simulink model "EnvironmentalControlSystem"  (R2018b)
settings: Solver=FixedStepAuto  StartTime=0.0  StopTime=500  FixedStep=0.01  RelTol=1e-3
values from neighbouring files (symbols this model uses):
  dt = 0.01    [run_sim.m]    (also in sys_id_pipeline.m = mean(diff(Time_vec_full)))
  K31 = Result31.K_slope    [sys_id_pipeline.m]
  K32 = Result32.K_slope    [sys_id_pipeline.m]
  P_ref = GlobalParams.P_ref    [sys_id_pipeline.m]
  Patm = GlobalParams.Patm    [sys_id_pipeline.m]
  R_gas = GlobalParams.R    [sys_id_pipeline.m]
  T_ref = GlobalParams.T_ref    [sys_id_pipeline.m]
  Tau31 = 5    [sys_id_pipeline.m]
  Tau32 = 5    [sys_id_pipeline.m]
  Tp31 = Result31.Tp    [sys_id_pipeline.m]
  Tp32 = Result32.Tp    [sys_id_pipeline.m]
  V_vol = pi * (0.05)^2 * 5    (= 0.0392699081699)    [run_sim.m]
  X31_den = sys_X31.Denominator    [sys_id_value.m]
  X31_num = sys_X31.Numerator    [sys_id_value.m]
  X32_den = sys_X32.Denominator    [sys_id_value.m]
  X32_num = sys_X32.Numerator    [sys_id_value.m]
libraries: simulink x14
(part 3 of 3)

== matlab function EnvironmentalControlSystem/ECS Controller/Smith_PI_Controller/Smith_PI_Controller ==
  settings: updateMethod=DISCRETE
  data: Q31Ref input; V31 output; Q31Real input; Q32Ref input; Q32Real input; P30 input; T30 input; V32 output; K31 parameter; Tau31 parameter; K32 parameter; Tau32 parameter; P_ref parameter; T_ref parameter; R_gas parameter; Patm parameter; X31_num parameter; X31_den parameter; X32_num parameter; Tp31 parameter; X32_den parameter; Tp32 parameter
function [V31, V32] = Smith_PI_Controller(Q31Ref, Q31Real, Q32Ref, Q32Real, P30, T30, K31, Tau31, K32, Tau32, P_ref, T_ref, R_gas, Patm, X31_num, X31_den, X32_num, Tp31, X32_den, Tp32)
    % Smith_PI_Controller_Optimized
    %
    % 本函数实现了一种针对双通道非线性流量控制系统的优化 Smith 预估 PI 控制策略。
    % 针对两路子系统（Q31和Q32）显著不同的动态特性（过阻尼 vs 欠阻尼）以及共同存在的
    % 执行器死区（Actuator Deadzone）和纯滞后（Pure Time Delay）问题，
    % 采用了差异化的控制律设计。核心算法集成了基于内部模型的 Smith 预估器以补偿滞后，
    % 并引入了动态软死区补偿（Soft Deadzone Compensation）、抗积分饱和（Anti-windup）
    % 以及软件误差死区（Software Error Deadband）机制，以解决响应迟滞和极限环震荡（Limit Cycle Oscillation）问题。
    %
    % 系统特性描述 (System Characterization):
    % 1. 通道 Q31 (过阻尼 Over-damped):
    %    - 特性：大惯性，响应迟钝，存在显著静摩擦。
    %    - 问题：起步困难，稳态易受死区补偿过度影响产生等幅震荡。
    %    - 策略：采用高增益 Smith-PI 进行快速驱动，结合带锁存功能的软死区补偿，以及较宽的误差死区来抑制稳态打桩效应。
    %
    % 2. 通道 Q32 (欠阻尼 Under-damped):
    %    - 特性：响应灵敏，阻尼比小，易超调。
    %    - 问题：系统本身接近临界稳定，易诱发高频震荡和极限环。
    %    - 策略：采用低增益控制，配合强效的软件误差死区，在稳态时切断积分作用，消除震荡源。
    %
    % 输入变量定义 (Input Variables):
    %   Q31Ref, Q32Ref : 流量设定值 (Reference Setpoint) [kg/h]
    %   Q31Real, Q32Real: 流量过程变量 (Process Variable) [kg/h]
    %   P30            : 上游压力 (Upstream Pressure) [kPa]
    %   T30            : 上游温度 (Upstream Temperature) [degC]
    %   [模型参数]      : K(静态增益), Tau(纯滞后), X_num/den(阀门传递函数系数), Tp(时间常数)
    %
    % 输出变量定义 (Output Variables):
    %   V31, V32       : 阀门控制指令 (Control Variable) [0-100%]

    % === 1. 状态记忆区 (Persistent State Memory) ===
    % 用于离散时间控制系统的状态保持
    
    persistent integrator_31 integrator_32  % PI控制器积分项累加器
    persistent model_31 model_32            % 内部快速模型状态向量 [阀位 x1; 阀速 x2; 流量 x3]
    persistent delay_buffer_31 delay_buffer_32 % 环形缓冲区，用于模拟纯滞后 Tau
    persistent head_31 head_32              % 环形缓冲区写指针
    persistent u_prev_31 u_prev_32          % 上一控制周期的输出指令 (用于差分计算)
    persistent first_run                    % 初始化标志位
    
    MAX_BUF = 1000; % 缓冲区最大长度 (支持的最大滞后步数)

    % === 系统初始化 (System Initialization) ===
    if isempty(first_run)
        integrator_31 = 0; integrator_32 = 0;
        model_31 = [0;0;0]; model_32 = [0;0;0];
        delay_buffer_31 = zeros(MAX_BUF, 1);
        delay_buffer_32 = zeros(MAX_BUF, 1);
        head_31 = 1; head_32 = 1;
        u_prev_31 = 0; u_prev_32 = 0;
        first_run = 0;
    end

    % === 2. 全局参数设定 (Global Parameters) ===
    Ts = 0.01; % 采样周期 (Sample Time) [s]
    
    % 增益调度因子计算 (Gain Scheduling Factor)
    % 依据流体力学原理，流量与压差平方根成正比。通过 Ratio 归一化过程增益，
    % 使得控制器在不同工况下保持一致的环路增益。
    Ratio = CalculateFlowRatio(P30, T30, P_ref, T_ref, R_gas, Patm);

    % ==========================================================
    %       控制策略配置 (CONTROL STRATEGY CONFIGURATION)
    % ==========================================================

    % --- 通道 31 配置 (针对过阻尼系统) ---
    % 策略逻辑：
    % 1. Kp_31 (1.8): 设置较高比例增益。Smith 预估器消除了滞后导致的相位滞后，允许提高带宽以克服过阻尼系统的惯性。
    % 2. Ti_31 (2.5): 增大积分时间常数。减弱积分作用，防止积分器在死区边缘过度充能，导致系统在目标值附近反复超调。
    % 3. Gap_31 (1.4): 适中的死区补偿值。用于在指令变化时提供额外的“启动脉冲”，克服静摩擦力。
    % 4. Err_Band_31 (0.6): 较宽的误差死区。这是消除稳态等幅震荡（Limit Cycle）的关键。当误差进入此范围，控制器停止调节，避免微小扰动触发死区补偿。
    Kp_31 = 1.8;  
    Ti_31 = 25;  
    Gap_31 = 1.4; 
    Err_Band_31 = 0.6; 

    % --- 通道 32 配置 (针对欠阻尼系统) ---
    % 策略逻辑：
    % 1. Kp_32 (0.3): 设置较低比例增益。欠阻尼系统对激励敏感，高增益极易激发系统固有频率震荡。
    % 2. Ti_32 (5.0): 极大的积分时间常数。微弱的积分作用仅用于消除长期静差，防止诱发过冲。
    % 3. Gap_32 (0.6): 较小的死区补偿。欠阻尼系统惯性小，无需强力启动，过大补偿会导致响应过激。
    % 4. Err_Band_32 (0.8): 宽误差死区。欠阻尼系统难以精确稳定在零误差，宽死区相当于提供一个“稳定停泊区”，切断极限环。
    Kp_32 = 0.3;  
    Ti_32 = 8.0;  
    Gap_32 = 0.6; 
    Err_Band_32 = 0.1; 

    % ==========================================================

    % --- 自适应控制参数计算 (Adaptive Parameter Calculation) ---
    % 根据当前的物理工况 (Ratio) 实时调整 PI 参数
    Ki_31 = Kp_31 / Ti_31;
    Kp_31_adpt = Kp_31 / Ratio;
    Ki_31_adpt = Ki_31 / Ratio;
    
    Ki_32 = Kp_32 / Ti_32;
    Kp_32_adpt = Kp_32 / Ratio;
    Ki_32_adpt = Ki_32 / Ratio;

    % ==========================================================
    %       通道 31 控制回路执行 (Control Loop Execution - Ch31)
    % ==========================================================
    
    % 1. Smith 预估器模型更新
    % 这里的模型不包含纯滞后，用于预测当前的“虚拟”无滞后响应。
    [model_31, Y_fast_31] = UpdateFastModel(model_31, u_prev_31, X31_num, X31_den, K31, Ratio, Tp31, Ts);
    
    % 2. 滞后环节模拟
    % 将无滞后响应通过延时队列，得到模型预测的有滞后响应。
    [delay_buffer_31, head_31, Y_delayed_31] = UpdateDelayBuffer(delay_buffer_31, head_31, Y_fast_31, Tau31, Ts, MAX_BUF);
    
    % 3. 模型失配补偿 (Model Mismatch Compensation)
    % 计算真实过程与模型预测之间的偏差（包含建模误差和外部干扰）。
    pred_error_31 = Q31Real - Y_delayed_31;
    
    % 4. 构造反馈主变量 (Process Variable Construction)
    % Smith 原理：反馈信号 = 无滞后模型输出 + 模型预测误差
    % 这使得主控制器感知到的对象是一个无滞后的传递函数 G(s)。
    PV_31 = Y_fast_31 + pred_error_31;
    
    % 5. 运行高级 PI 控制算法
    [u_raw_31, integrator_31, error_31] = RunPI(Q31Ref, PV_31, integrator_31, Kp_31_adpt, Ki_31_adpt, Ts, Err_Band_31);
    
    % 6. 应用带锁存功能的软死区补偿
    % 针对 31 路，增加锁存阈值至 1.5，以平滑补偿动作。
    V31 = InverseDeadzoneComp_Soft(u_raw_31, u_prev_31, Gap_31, error_31, 1.5); 
    
    u_prev_31 = V31; % 状态更新

    % ==========================================================
    %       通道 32 控制回路执行 (Control Loop Execution - Ch32)
    % ==========================================================
    
    % 步骤同上，应用针对欠阻尼系统的参数集
    [model_32, Y_fast_32] = UpdateFastModel(model_32, u_prev_32, X32_num, X32_den, K32, Ratio, Tp32, Ts);
    [delay_buffer_32, head_32, Y_delayed_32] = UpdateDelayBuffer(delay_buffer_32, head_32, Y_fast_32, Tau32, Ts, MAX_BUF);
    
    pred_error_32 = Q32Real - Y_delayed_32;
    PV_32 = Y_fast_32 + pred_error_32;
    
    [u_raw_32, integrator_32, error_32] = RunPI(Q32Ref, PV_32, integrator_32, Kp_32_adpt, Ki_32_adpt, Ts, Err_Band_32);
    
    % 32路死区补偿：使用默认阈值 1.0
    V32 = InverseDeadzoneComp_Soft(u_raw_32, u_prev_32, Gap_32, error_32, 1.0);
    
    u_prev_32 = V32;
end

%% === 核心模块 1: 高级 PI 控制器 (Advanced PI Controller) ===
% 功能：实现比例-积分控制律，集成了抗积分饱和与误差死区功能。
function [u_out, I_new, eff_err] = RunPI(Ref, Meas, I_old, Kp, Ki, Ts, ErrDeadband)
    raw_error = Ref - Meas;
    
    % --- 软件误差死区逻辑 (Software Error Deadband Logic) ---
    % 目的：消除稳态极限环震荡。
    % 原理：当误差小于预设阈值时，强制认为系统已收敛，切断误差信号。
    if abs(raw_error) < ErrDeadband
        effective_error = 0; % 有效误差置零
        I_new = I_old;       % 积分器保持（冻结）
        u_out = I_old;       % 输出保持上一时刻积分值（此时 P 项为 0）
        eff_err = 0; 
        return; 
    else
        effective_error = raw_error;
    end
    
    % --- PI 计算 ---
    P_term = Kp * effective_error;
    I_temp = I_old + Ki * effective_error * Ts; % 预积分
    u_temp = P_term + I_temp;
    
    % --- 抗积分饱和逻辑 (Anti-windup Logic - Clamping Method) ---
    % 目的：防止执行器饱和时积分器持续累积导致退饱和滞后。
    % 逻辑：当计算输出超出物理限制时，如果误差方向未能使系统退出饱和，则冻结积分器。
    if u_temp > 100
        u_out = 100;
        if effective_error > 0, I_new = I_old; else, I_new = I_temp; end
    elseif u_temp < 0
        u_out = 0;
        if effective_error < 0, I_new = I_old; else, I_new = I_temp; end
    else
        u_out = u_temp;
        I_new = I_temp;
    end
    eff_err = effective_error;
end

%% === 核心模块 2: 软死区补偿与输出锁存 (Soft Compensation & Output Latch) ===
% 功能：补偿执行器死区特性，并引入平滑机制防止控制指令跳变震荡。
function u_final = InverseDeadzoneComp_Soft(u_cmd, u_last, gap, error, err_threshold)
    delta = u_cmd - u_last;
    
    % --- 动态补偿系数 (Dynamic Compensation Factor) ---
    % 目的：实现补偿力度的渐进式变化。
    % 算法：根据当前跟踪误差的大小线性调整补偿量。误差大时全额补偿，误差小时减弱补偿。
    alpha = min(abs(error) / err_threshold, 1.0);
    real_gap = gap * alpha;
    
    % --- 输出锁存逻辑 (Output Latch Logic) ---
    % 目的：消除微小指令变化引起的震荡。
    % 逻辑：设定噪声门限 (Noise_Threshold)。若指令增量小于此门限，视为无效抖动，
    % 强制保持上一时刻输出不变。这有效防止了补偿器在临界点频繁开关。
    Noise_Threshold = 0.02; 
    
    if abs(delta) > Noise_Threshold 
        if delta > 0
            u_final = u_cmd + real_gap; % 正向补偿
        else
            u_final = u_cmd - real_gap; % 反向补偿
        end
    else
        u_final = u_last; % 锁存输出
    end
    
    % 物理限幅
    u_final = max(0, min(100, u_final));
end

%% === 辅助模块 3: 快速模型更新 (Fast Model Update) ===
% 功能：基于离散化状态空间方程，模拟无滞后的系统动态。
function [state_new, y_flow] = UpdateFastModel(state, u_in, num, den, K, Ratio, Tp, Ts)
    wn2 = den(3); zw = den(2); K_valve = num; K_total = K * Ratio;
    x1 = state(1); x2 = state(2); x3 = state(3);
    
    % 阀门二阶动力学 (Euler 积分)
    acc = K_valve * u_in - zw * x2 - wn2 * x1;
    x2_new = x2 + acc * Ts;
    x1_new = x1 + x2 * Ts;
    
    % 管道一阶流体动力学
    dy = (K_total * x1 - x3) / max(Tp, 0.1);
    x3_new = x3 + dy * Ts;
    
    state_new = [x1_new; x2_new; x3_new];
    y_flow = x3_new;
end

%% === 辅助模块 4: 延时队列管理 (Delay Buffer Management) ===
% 功能：使用环形缓冲区实现固定步长的纯滞后模拟。
function [buffer, head_idx, y_delayed] = UpdateDelayBuffer(buffer, head, y_in, Tau, Ts, MAX_BUF)
    delay_steps = round(Tau / Ts);
    delay_steps = max(1, min(delay_steps, MAX_BUF - 1));
    buffer(head) = y_in;
    read_idx = head - delay_steps;
    if read_idx < 1, read_idx = read_idx + MAX_BUF; end
    y_delayed = buffer(read_idx);
    head_idx = head + 1;
    if head_idx > MAX_BUF, head_idx = 1; end
end

%% === 辅助模块 5: 物理增益计算 (Physical Gain Calculation) ===
% 功能：基于理想气体流动方程计算流量修正系数。
function Ratio = CalculateFlowRatio(P30, T30, P_ref, T_ref, R_gas, Patm)
    Tk_dyn = T30 + 273.15; delta_P_dyn = P30 - Patm;
    if delta_P_dyn < 0, delta_P_dyn = 0; end
    Term_Dyn = sqrt((P30 * 1000 * delta_P_dyn * 1000) / (R_gas * Tk_dyn));
    Tk_ref = T_ref + 273.15; delta_P_ref = P_ref - Patm;
    if delta_P_ref < 0, delta_P_ref = 0; end
    Term_Ref = sqrt((P_ref * 1000 * delta_P_ref * 1000) / (R_gas * Tk_ref));
    if Term_Ref < 1e-6, Ratio = 1; else, Ratio = max(Term_Dyn / Term_Ref, 0.05); end
end

== matlab function EnvironmentalControlSystem/ECS Controller/Simple Controller/PID_Controller/Air Conditioning Value/X31Deadband ==
  data: curPos input; u_eff output; cmdPos input
function u_eff = X31Deadband(curPos, cmdPos)
    % 引入持久变量来记录系统当前的状态：是在"调节中"还是"已到位"
    persistent isAdjusting
    if isempty(isAdjusting)
        isAdjusting = false;
    end

    % === 参数设置 ===
    % Start_Deadband: 启动死区（防抖阈值）。误差超过此值，开始动作
    % 设为 3，意味着噪声在 +/-3 以内时，若系统本来是静止的，就不理会
    Start_Deadband = 2.0; 
    
    % Stop_Deadband: 停止死区（精度阈值）。误差小于此值，才算到位
    % 设为 0.5，意味着一旦动起来，必须修到 99.5~100.5 之间才停手
    Stop_Deadband  = 0.2; 

    % 计算当前误差绝对值
    err = abs(cmdPos - curPos);

    % === 状态机逻辑 ===
    if isAdjusting
        % 【状态1：正在调节中】
        % 既然已经动起来了，就要追求高精度。
        % 只有当误差足够小（满足精度要求）时，才停止。
        if err <= Stop_Deadband
            isAdjusting = false; % 切换状态：认为已到位
            u_eff = curPos;      % 欺骗控制器误差为0，使其停止积分/输出
        else
            isAdjusting = true;  % 保持调节状态
            u_eff = cmdPos;      % 正常输出目标值给控制器
        end
    else
        % 【状态2：已到位/静止中】
        % 此时为了防抖，对小误差视而不见。
        % 只有当误差突然变大（超过启动阈值，比如新指令来了）时，才开始动
        if err > Start_Deadband
            isAdjusting = true;  % 切换状态：开始调节
            u_eff = cmdPos;      % 输出目标值
        else
            isAdjusting = false; % 保持静止
            u_eff = curPos;      % 锁定当前位置，抑制抖动
        end
    end
end

== matlab function EnvironmentalControlSystem/ECS Controller/Simple Controller/PID_Controller/Anti-icing Pipeline /MATLAB Function ==
  data: X input; Q_static output; P30 input; T30 input; K32 parameter; P_ref parameter; T_ref parameter; R_gas parameter; Patm parameter
function Q_static = StaticCalc(X, P30, T30, K32, P_ref, T_ref, R_gas, Patm)
    % 输入单位说明:
    % X: 阀门开度 (0-1 或 0-100，取决于你的K是基于什么单位)
    % P_dyn: 实时压力 (kPa)
    % T_dyn: 实时温度 (摄氏度)
    
    % --- 1. 计算标称流量 (Nominal Flow) ---
    Q_nominal = K32 * X;
    
    % --- 2. 计算实时物理因子 (Real-time Term) ---
    % 温度转开尔文
    Tk_dyn = T30 + 273.15;
    delta_P_dyn = P30 - Patm;
    Term_Dyn = sqrt(max((P30 * delta_P_dyn) / (R_gas * Tk_dyn), 0));
    
    % --- 3. 计算参考物理因子 (Reference Term - Constant) ---
    Tk_ref = T_ref + 273.15;
    delta_P_ref = P_ref - Patm;
    Term_Ref = sqrt(max((P_ref * delta_P_ref) / (R_gas * Tk_ref), 0));
    
    % --- 4. 计算最终静态流量 ---
    if Term_Ref < 1e-6
        Ratio = 1;
    else
        Ratio = Term_Dyn / Term_Ref;
    end
    
    Q_static = Q_nominal * Ratio;
end

== matlab function EnvironmentalControlSystem/ECS Controller/Simple Controller/PID_Controller/Anti-icing Value/X32Deadband ==
  data: curPos input; u_eff output; cmdPos input
function u_eff = X32Deadband(curPos, cmdPos)
    % 引入持久变量来记录系统当前的状态：是在"调节中"还是"已到位"
    persistent isAdjusting
    if isempty(isAdjusting)
        isAdjusting = false;
    end

    % === 参数设置 ===
    % Start_Deadband: 启动死区（防抖阈值）。误差超过此值，开始动作
    % 设为 3，意味着噪声在 +/-3 以内时，若系统本来是静止的，就不理会
    Start_Deadband = 2.0; 
    
    % Stop_Deadband: 停止死区（精度阈值）。误差小于此值，才算到位
    % 设为 0.5，意味着一旦动起来，必须修到 99.5~100.5 之间才停手
    Stop_Deadband  = 0.2; 

    % 计算当前误差绝对值
    err = abs(cmdPos - curPos);

    % === 状态机逻辑 ===
    if isAdjusting
        % 【状态1：正在调节中】
        % 既然已经动起来了，就要追求高精度。
        % 只有当误差足够小（满足精度要求）时，才停止。
        if err <= Stop_Deadband
            isAdjusting = false; % 切换状态：认为已到位
            u_eff = curPos;      % 欺骗控制器误差为0，使其停止积分/输出
        else
            isAdjusting = true;  % 保持调节状态
            u_eff = cmdPos;      % 正常输出目标值给控制器
        end
    else
        % 【状态2：已到位/静止中】
        % 此时为了防抖，对小误差视而不见。
        % 只有当误差突然变大（超过启动阈值，比如新指令来了）时，才开始动
        if err > Start_Deadband
            isAdjusting = true;  % 切换状态：开始调节
            u_eff = cmdPos;      % 输出目标值
        else
            isAdjusting = false; % 保持静止
            u_eff = curPos;      % 锁定当前位置，抑制抖动
        end
    end
end

== matlab function EnvironmentalControlSystem/ECS Controller/Simple Controller/Smith_PI_Controller/Air Conditioning Pipeline/MATLAB Function ==
  data: X input; Q_static output; P30 input; T30 input; K31 parameter; P_ref parameter; T_ref parameter; R_gas parameter; Patm parameter
function Q_static = StaticCalc(X, P30, T30, K31, P_ref, T_ref, R_gas, Patm)
    % 输入单位说明:
    % X: 阀门开度 (0-1 或 0-100，取决于你的K是基于什么单位)
    % P_dyn: 实时压力 (kPa)
    % T_dyn: 实时温度 (摄氏度)
    
    % --- 1. 计算标称流量 (Nominal Flow) ---
    Q_nominal = K31 * X;
    
    % --- 2. 计算实时物理因子 (Real-time Term) ---
    % 温度转开尔文
    Tk_dyn = T30 + 273.15;
    delta_P_dyn = P30 - Patm;
    Term_Dyn = sqrt(max((P30 * delta_P_dyn) / (R_gas * Tk_dyn), 0));
    
    % --- 3. 计算参考物理因子 (Reference Term - Constant) ---
    Tk_ref = T_ref + 273.15;
    delta_P_ref = P_ref - Patm;
    Term_Ref = sqrt(max((P_ref * delta_P_ref) / (R_gas * Tk_ref), 0));
    
    % --- 4. 计算最终静态流量 (修正后) ---
    if Term_Ref < 1e-6
        Ratio = 1;
    else
        Ratio = Term_Dyn / Term_Ref;
    end
    
    Q_static = Q_nominal * Ratio;
end

== matlab function EnvironmentalControlSystem/ECS Controller/Simple Controller/Smith_PI_Controller/Air Conditioning Value/X31Deadband ==
  data: curPos input; u_eff output; cmdPos input
function u_eff = X31Deadband(curPos, cmdPos)
    % 引入持久变量来记录系统当前的状态：是在"调节中"还是"已到位"
    persistent isAdjusting
    if isempty(isAdjusting)
        isAdjusting = false;
    end

    % === 参数设置 ===
    % Start_Deadband: 启动死区（防抖阈值）。误差超过此值，开始动作
    % 设为 3，意味着噪声在 +/-3 以内时，若系统本来是静止的，就不理会
    Start_Deadband = 2.0; 
    
    % Stop_Deadband: 停止死区（精度阈值）。误差小于此值，才算到位
    % 设为 0.5，意味着一旦动起来，必须修到 99.5~100.5 之间才停手
    Stop_Deadband  = 0.2; 

    % 计算当前误差绝对值
    err = abs(cmdPos - curPos);

    % === 状态机逻辑 ===
    if isAdjusting
        % 【状态1：正在调节中】
        % 既然已经动起来了，就要追求高精度。
        % 只有当误差足够小（满足精度要求）时，才停止。
        if err <= Stop_Deadband
            isAdjusting = false; % 切换状态：认为已到位
            u_eff = curPos;      % 欺骗控制器误差为0，使其停止积分/输出
        else
            isAdjusting = true;  % 保持调节状态
            u_eff = cmdPos;      % 正常输出目标值给控制器
        end
    else
        % 【状态2：已到位/静止中】
        % 此时为了防抖，对小误差视而不见。
        % 只有当误差突然变大（超过启动阈值，比如新指令来了）时，才开始动
        if err > Start_Deadband
            isAdjusting = true;  % 切换状态：开始调节
            u_eff = cmdPos;      % 输出目标值
        else
            isAdjusting = false; % 保持静止
            u_eff = curPos;      % 锁定当前位置，抑制抖动
        end
    end
end

== matlab function EnvironmentalControlSystem/ECS Controller/Simple Controller/Smith_PI_Controller/Anti-icing Pipeline /MATLAB Function ==
  data: X input; Q_static output; P30 input; T30 input; K32 parameter; P_ref parameter; T_ref parameter; R_gas parameter; Patm parameter
function Q_static = StaticCalc(X, P30, T30, K32, P_ref, T_ref, R_gas, Patm)
    % 输入单位说明:
    % X: 阀门开度 (0-1 或 0-100，取决于你的K是基于什么单位)
    % P_dyn: 实时压力 (kPa)
    % T_dyn: 实时温度 (摄氏度)
    
    % --- 1. 计算标称流量 (Nominal Flow) ---
    Q_nominal = K32 * X;
    
    % --- 2. 计算实时物理因子 (Real-time Term) ---
    % 温度转开尔文
    Tk_dyn = T30 + 273.15;
    delta_P_dyn = P30 - Patm;
    Term_Dyn = sqrt(max((P30 * delta_P_dyn) / (R_gas * Tk_dyn), 0));
    
    % --- 3. 计算参考物理因子 (Reference Term - Constant) ---
    Tk_ref = T_ref + 273.15;
    delta_P_ref = P_ref - Patm;
    Term_Ref = sqrt(max((P_ref * delta_P_ref) / (R_gas * Tk_ref), 0));
    
    % --- 4. 计算最终静态流量 ---
    if Term_Ref < 1e-6
        Ratio = 1;
    else
        Ratio = Term_Dyn / Term_Ref;
    end
    
    Q_static = Q_nominal * Ratio;
end

== matlab function EnvironmentalControlSystem/ECS Controller/Simple Controller/Smith_PI_Controller/Anti-icing Value/X32Deadband ==
  data: curPos input; u_eff output; cmdPos input
function u_eff = X32Deadband(curPos, cmdPos)
    % 引入持久变量来记录系统当前的状态：是在"调节中"还是"已到位"
    persistent isAdjusting
    if isempty(isAdjusting)
        isAdjusting = false;
    end

    % === 参数设置 ===
    % Start_Deadband: 启动死区（防抖阈值）。误差超过此值，开始动作
    % 设为 3，意味着噪声在 +/-3 以内时，若系统本来是静止的，就不理会
    Start_Deadband = 2.0; 
    
    % Stop_Deadband: 停止死区（精度阈值）。误差小于此值，才算到位
    % 设为 0.5，意味着一旦动起来，必须修到 99.5~100.5 之间才停手
    Stop_Deadband  = 0.2; 

    % 计算当前误差绝对值
    err = abs(cmdPos - curPos);

    % === 状态机逻辑 ===
    if isAdjusting
        % 【状态1：正在调节中】
        % 既然已经动起来了，就要追求高精度。
        % 只有当误差足够小（满足精度要求）时，才停止。
        if err <= Stop_Deadband
            isAdjusting = false; % 切换状态：认为已到位
            u_eff = curPos;      % 欺骗控制器误差为0，使其停止积分/输出
        else
            isAdjusting = true;  % 保持调节状态
            u_eff = cmdPos;      % 正常输出目标值给控制器
        end
    else
        % 【状态2：已到位/静止中】
        % 此时为了防抖，对小误差视而不见。
        % 只有当误差突然变大（超过启动阈值，比如新指令来了）时，才开始动
        if err > Start_Deadband
            isAdjusting = true;  % 切换状态：开始调节
            u_eff = cmdPos;      % 输出目标值
        else
            isAdjusting = false; % 保持静止
            u_eff = curPos;      % 锁定当前位置，抑制抖动
        end
    end
end

== matlab function EnvironmentalControlSystem/ECS Controller/Simple Controller/Smith_PI_Controller/Q31Controller ==
  settings: updateMethod=DISCRETE
  data: Q31Ref input; V31 output; Q31Real input; P30 input; T30 input; K31 parameter; Tau31 parameter; K32 parameter; Tau32 parameter; P_ref parameter; T_ref parameter; R_gas parameter; Patm parameter; X31_num parameter; X31_den parameter; X32_num parameter; Tp31 parameter; X32_den parameter; Tp32 parameter; dt parameter
function V31  = Smith_PI_Controller(Q31Ref, Q31Real, P30, T30, K31, Tau31, K32, Tau32, P_ref, T_ref, R_gas, Patm, X31_num, X31_den, X32_num, Tp31, X32_den, Tp32, dt)
    % Smith_PI_Controller_Optimized
    %
    % 本函数实现了一种针对双通道非线性流量控制系统的优化 Smith 预估 PI 控制策略。
    % 针对两路子系统（Q31和Q32）显著不同的动态特性（过阻尼 vs 欠阻尼）以及共同存在的
    % 执行器死区（Actuator Deadzone）和纯滞后（Pure Time Delay）问题，
    % 采用了差异化的控制律设计。核心算法集成了基于内部模型的 Smith 预估器以补偿滞后，
    % 并引入了动态软死区补偿（Soft Deadzone Compensation）、抗积分饱和（Anti-windup）
    % 以及软件误差死区（Software Error Deadband）机制，以解决响应迟滞和极限环震荡（Limit Cycle Oscillation）问题。
    %
    % 系统特性描述 (System Characterization):
    % 1. 通道 Q31 (过阻尼 Over-damped):
    %    - 特性：大惯性，响应迟钝，存在显著静摩擦。
    %    - 问题：起步困难，稳态易受死区补偿过度影响产生等幅震荡。
    %    - 策略：采用高增益 Smith-PI 进行快速驱动，结合带锁存功能的软死区补偿，以及较宽的误差死区来抑制稳态打桩效应。
    %
    % 2. 通道 Q32 (欠阻尼 Under-damped):
    %    - 特性：响应灵敏，阻尼比小，易超调。
    %    - 问题：系统本身接近临界稳定，易诱发高频震荡和极限环。
    %    - 策略：采用低增益控制，配合强效的软件误差死区，在稳态时切断积分作用，消除震荡源。
    %
    % 输入变量定义 (Input Variables):
    %   Q31Ref, Q32Ref : 流量设定值 (Reference Setpoint) [kg/h]
    %   Q31Real, Q32Real: 流量过程变量 (Process Variable) [kg/h]
    %   P30            : 上游压力 (Upstream Pressure) [kPa]
    %   T30            : 上游温度 (Upstream Temperature) [degC]
    %   [模型参数]      : K(静态增益), Tau(纯滞后), X_num/den(阀门传递函数系数), Tp(时间常数)
    %
    % 输出变量定义 (Output Variables):
    %   V31, V32       : 阀门控制指令 (Control Variable) [0-100%]

    % === 1. 状态记忆区 (Persistent State Memory) ===
    % 用于离散时间控制系统的状态保持
    
    persistent integrator_31        % PI控制器积分项累加器
    persistent model_31             % 内部快速模型状态向量 [阀位 x1; 阀速 x2; 流量 x3]
    persistent delay_buffer_31      % 环形缓冲区，用于模拟纯滞后 Tau
    persistent head_31              % 环形缓冲区写指针
    persistent u_prev_31            % 上一控制周期的输出指令 (用于差分计算)
    persistent first_run            % 初始化标志位
    
    MAX_BUF = 1000; % 缓冲区最大长度 (支持的最大滞后步数)

    % === 系统初始化 (System Initialization) ===
    if isempty(first_run)
        integrator_31 = 0;
        model_31 = [0;0;0];
        delay_buffer_31 = zeros(MAX_BUF, 1);
        head_31 = 1;
        u_prev_31 = 0;
        first_run = 0;
    end

    % === 2. 全局参数设定 (Global Parameters) ===
    
    % 增益调度因子计算 (Gain Scheduling Factor)
    % 依据流体力学原理，流量与压差平方根成正比。通过 Ratio 归一化过程增益，
    % 使得控制器在不同工况下保持一致的环路增益。
    Ratio = CalculateFlowRatio(P30, T30, P_ref, T_ref, R_gas, Patm);

    % ==========================================================
    %       控制策略配置 (CONTROL STRATEGY CONFIGURATION)
    % ==========================================================

    % --- 通道 31 配置 (针对过阻尼系统) ---
    % 策略逻辑：
    % 1. Kp_31 (1.8): 设置较高比例增益。Smith 预估器消除了滞后导致的相位滞后，允许提高带宽以克服过阻尼系统的惯性。
    % 2. Ti_31 (2.5): 增大积分时间常数。减弱积分作用，防止积分器在死区边缘过度充能，导致系统在目标值附近反复超调。
    % 3. Gap_31 (1.4): 适中的死区补偿值。用于在指令变化时提供额外的“启动脉冲”，克服静摩擦力。
    % 4. Err_Band_31 (0.6): 较宽的误差死区。这是消除稳态等幅震荡（Limit Cycle）的关键。当误差进入此范围，控制器停止调节，避免微小扰动触发死区补偿。
    Kp_31 = 1.8;  
    Ti_31 = 25;  
    Gap_31 = 1.4; 
    Err_Band_31 = 0.6; 

    % ==========================================================

    % --- 自适应控制参数计算 (Adaptive Parameter Calculation) ---
    % 根据当前的物理工况 (Ratio) 实时调整 PI 参数
    Ki_31 = Kp_31 / Ti_31;
    Kp_31_adpt = Kp_31 / Ratio;
    Ki_31_adpt = Ki_31 / Ratio;
    

    % ==========================================================
    %       通道 31 控制回路执行 (Control Loop Execution - Ch31)
    % ==========================================================
    
    % 1. Smith 预估器模型更新
    % 这里的模型不包含纯滞后，用于预测当前的“虚拟”无滞后响应。
    [model_31, Y_fast_31] = UpdateFastModel(model_31, u_prev_31, X31_num, X31_den, K31, Ratio, Tp31, dt);
    
    % 2. 滞后环节模拟
    % 将无滞后响应通过延时队列，得到模型预测的有滞后响应。
    [delay_buffer_31, head_31, Y_delayed_31] = UpdateDelayBuffer(delay_buffer_31, head_31, Y_fast_31, Tau31, dt, MAX_BUF);
    
    % 3. 模型失配补偿 (Model Mismatch Compensation)
    % 计算真实过程与模型预测之间的偏差（包含建模误差和外部干扰）。
    pred_error_31 = Q31Real - Y_delayed_31;
    
    % 4. 构造反馈主变量 (Process Variable Construction)
    % Smith 原理：反馈信号 = 无滞后模型输出 + 模型预测误差
    % 这使得主控制器感知到的对象是一个无滞后的传递函数 G(s)。
    PV_31 = Y_fast_31 + pred_error_31;
    
    % 5. 运行高级 PI 控制算法
    [u_raw_31, integrator_31, error_31] = RunPI(Q31Ref, PV_31, integrator_31, Kp_31_adpt, Ki_31_adpt, dt, Err_Band_31);
    
    % 6. 应用带锁存功能的软死区补偿
    % 针对 31 路，增加锁存阈值至 1.5，以平滑补偿动作。
    V31 = InverseDeadzoneComp_Soft31(u_raw_31, u_prev_31, Gap_31, error_31, 1.5); 
    
    u_prev_31 = V31; % 状态更新
end

%% === 核心模块 1: 高级 PI 控制器 (Advanced PI Controller) ===
% 功能：实现比例-积分控制律，集成了抗积分饱和与误差死区功能。
function [u_out, I_new, eff_err] = RunPI(Ref, Meas, I_old, Kp, Ki, Ts, ErrDeadband)
    raw_error = Ref - Meas;
    
    % --- 软件误差死区逻辑 (Software Error Deadband Logic) ---
    % 目的：消除稳态极限环震荡
    % 原理：当误差小于预设阈值时，强制认为系统已收敛，切断误差信号
    if abs(raw_error) < ErrDeadband
        effective_error = 0; % 有效误差置零
        I_new = I_old;       % 积分器保持（冻结）
        u_out = I_old;       % 输出保持上一时刻积分值（此时 P 项为 0）
        eff_err = 0; 
        return; 
    else
        effective_error = raw_error;
    end
    
    % --- PI 计算 ---
    P_term = Kp * effective_error;
    I_temp = I_old + Ki * effective_error * Ts; % 预积分
    u_temp = P_term + I_temp;
    
    % --- 抗积分饱和逻辑 (Anti-windup Logic - Clamping Method) ---
    % 目的：防止执行器饱和时积分器持续累积导致退饱和滞后。
    % 逻辑：当计算输出超出物理限制时，如果误差方向未能使系统退出饱和，则冻结积分器。
    if u_temp > 100
        u_out = 100;
        if effective_error > 0, I_new = I_old; else, I_new = I_temp; end
    elseif u_temp < 0
        u_out = 0;
        if effective_error < 0, I_new = I_old; else, I_new = I_temp; end
    else
        u_out = u_temp;
        I_new = I_temp;
    end
    eff_err = effective_error;
end

%% === 核心模块 2: 软死区补偿与输出锁存 (Soft Compensation & Output Latch) ===
% 功能：补偿执行器死区特性，并引入平滑机制防止控制指令跳变震荡。
function u_final = InverseDeadzoneComp_Soft31(u_cmd, u_last, gap, error, err_threshold)
    delta = u_cmd - u_last;
    
    % --- 动态补偿系数 (Dynamic Compensation Factor) ---
    % 目的：实现补偿力度的渐进式变化
    % 算法：根据当前跟踪误差的大小线性调整补偿量。误差大时全额补偿，误差小时减弱补偿
    alpha = min(abs(error) / err_threshold, 1.0);
    real_gap = gap * alpha;
    
    % --- 输出锁存逻辑 (Output Latch Logic) ---
    % 目的：消除微小指令变化引起的震荡
    % 逻辑：设定噪声门限 (Noise_Threshold)。若指令增量小于此门限，视为无效抖动，
    % 强制保持上一时刻输出不变。这有效防止了补偿器在临界点频繁开关
    Noise_Threshold = 0.02; 
    
    if abs(delta) > Noise_Threshold 
        if delta > 0
            u_final = u_cmd + real_gap; % 正向补偿
        else
            u_final = u_cmd - real_gap; % 反向补偿
        end
    else
        u_final = u_last; % 锁存输出
    end
    
    % 物理限幅
    u_final = max(0, min(100, u_final));
end

%% === 辅助模块 3: 快速模型更新 (Fast Model Update) ===
% 功能：基于离散化状态空间方程，模拟无滞后的系统动态               
function [state_new, y_flow] = UpdateFastModel(state, u_in, num, den, K, Ratio, Tp, Ts)
    wn2 = den(3); zw = den(2); K_valve = num; K_total = K * Ratio;
    x1 = state(1); x2 = state(2); x3 = state(3);
    
    % 阀门二阶动力学 (Euler 积分)
    acc = K_valve * u_in - zw * x2 - wn2 * x1;
    x2_new = x2 + acc * Ts;
    x1_new = x1 + x2 * Ts;
    
    % 管道一阶流体动力学
    dy = (K_total * x1 - x3) / max(Tp, 0.1);
    x3_new = x3 + dy * Ts;
    
    state_new = [x1_new; x2_new; x3_new];
    y_flow = x3_new;
end

%% === 辅助模块 4: 延时队列管理 (Delay Buffer Management) ===
% 功能：使用环形缓冲区实现固定步长的纯滞后模拟
function [buffer, head_idx, y_delayed] = UpdateDelayBuffer(buffer, head, y_in, Tau, Ts, MAX_BUF)
    % 计算滞后步长
    delay_steps = round(Tau / Ts);
    delay_steps = max(1, min(delay_steps, MAX_BUF - 1));
    % 写入新数据
    buffer(head) = y_in;
    % 读取旧数据与处理环形逻辑
    read_idx = head - delay_steps;
    if read_idx < 1, read_idx = read_idx + MAX_BUF; end
    y_delayed = buffer(read_idx);
    % 更新指针
    head_idx = head + 1;
    if head_idx > MAX_BUF, head_idx = 1; end
end

%% === 辅助模块 5: 物理增益计算 (Physical Gain Calculation) ===
% 功能：基于理想气体流动方程计算流量修正系数
function Ratio = CalculateFlowRatio(P30, T30, P_ref, T_ref, R_gas, Patm)
    Tk_dyn = T30 + 273.15; delta_P_dyn = P30 - Patm;
    if delta_P_dyn < 0, delta_P_dyn = 0; end
    Term_Dyn = sqrt((P30 * 1000 * delta_P_dyn * 1000) / (R_gas * Tk_dyn));
    Tk_ref = T_ref + 273.15; delta_P_ref = P_ref - Patm;
    if delta_P_ref < 0, delta_P_ref = 0; end
    Term_Ref = sqrt((P_ref * 1000 * delta_P_ref * 1000) / (R_gas * Tk_ref));
    if Term_Ref < 1e-6, Ratio = 1; else, Ratio = max(Term_Dyn / Term_Ref, 0.05); end
end

== matlab function EnvironmentalControlSystem/ECS Controller/Simple Controller/Smith_iLQR_Controller/Anti-icing Value/X32Deadband ==
  data: curPos input; u_eff output; cmdPos input
function u_eff = X32Deadband(curPos, cmdPos)
    % 引入持久变量来记录系统当前的状态：是在"调节中"还是"已到位"
    persistent isAdjusting
    if isempty(isAdjusting)
        isAdjusting = false;
    end

    % === 参数设置 ===
    % Start_Deadband: 启动死区（防抖阈值）。误差超过此值，开始动作
    % 设为 3，意味着噪声在 +/-3 以内时，若系统本来是静止的，就不理会
    Start_Deadband = 2.0; 
    
    % Stop_Deadband: 停止死区（精度阈值）。误差小于此值，才算到位
    % 设为 0.5，意味着一旦动起来，必须修到 99.5~100.5 之间才停手
    Stop_Deadband  = 0.2; 

    % 计算当前误差绝对值
    err = abs(cmdPos - curPos);

    % === 状态机逻辑 ===
    if isAdjusting
        % 【状态1：正在调节中】
        % 既然已经动起来了，就要追求高精度。
        % 只有当误差足够小（满足精度要求）时，才停止。
        if err <= Stop_Deadband
            isAdjusting = false; % 切换状态：认为已到位
            u_eff = curPos;      % 欺骗控制器误差为0，使其停止积分/输出
        else
            isAdjusting = true;  % 保持调节状态
            u_eff = cmdPos;      % 正常输出目标值给控制器
        end
    else
        % 【状态2：已到位/静止中】
        % 此时为了防抖，对小误差视而不见。
        % 只有当误差突然变大（超过启动阈值，比如新指令来了）时，才开始动
        if err > Start_Deadband
            isAdjusting = true;  % 切换状态：开始调节
            u_eff = cmdPos;      % 输出目标值
        else
            isAdjusting = false; % 保持静止
            u_eff = curPos;      % 锁定当前位置，抑制抖动
        end
    end
end

== matlab function EnvironmentalControlSystem/ECS Controller/Simple Controller/Smith_iLQR_Controller/Smith_iLQR_Controller ==
  settings: updateMethod=DISCRETE
  data: Q31Ref input; V31 output; Q31Real input; Q32Ref input; Q32Real input; P30 input; T30 input; V32 output; K31 parameter; Tau31 parameter; K32 parameter; Tau32 parameter; P_ref parameter; T_ref parameter; R_gas parameter; Patm parameter; X31_num parameter; X31_den parameter; X32_num parameter; Tp31 parameter; X32_den parameter; Tp32 parameter; dt parameter
function [V31, V32] = Smith_iLQR_Integral_Controller(Q31Ref, Q31Real, Q32Ref, Q32Real, P30, T30, K31, Tau31, K32, Tau32, P_ref, T_ref, R_gas, Patm, X31_num, X31_den, X32_num, Tp31, X32_den, Tp32, dt)
    % Smith_iLQR_Integral_Controller
    %
    % 更新日志:
    % - [New] Q32 增加了自适应 R 权重 (Adaptive R) 策略。
    %   原理：大误差时关闭平滑惩罚(R=0)以求快；小误差时开启强平滑惩罚(R=20)以求稳。
    %
    % 核心思路:
    % 1. Smith 预估 + 积分型 iLQR (消除稳态误差)
    % 2. 状态扩充：x = [阀位; 阀速; 流量; 误差积分]

    persistent model_31 model_32            
    persistent delay_buffer_31 delay_buffer_32 
    persistent head_31 head_32              
    persistent u_prev_31 u_prev_32          
    persistent u_opt_guess_31 u_opt_guess_32 
    persistent x_int_31 x_int_32
    persistent first_run

    MAX_BUF = 1000; 
    HORIZON = 20; 

    if isempty(first_run)
        model_31 = [0;0;0]; model_32 = [0;0;0];
        x_int_31 = 0; x_int_32 = 0;
        
        delay_buffer_31 = zeros(MAX_BUF, 1);
        delay_buffer_32 = zeros(MAX_BUF, 1);
        head_31 = 1; head_32 = 1;
        u_prev_31 = 0; u_prev_32 = 0;
        u_opt_guess_31 = zeros(HORIZON, 1); 
        u_opt_guess_32 = zeros(HORIZON, 1);
        first_run = 0;
    end

    Ratio = CalculateFlowRatio(P30, T30, P_ref, T_ref, R_gas, Patm);

    % === 权重配置 ===
    
    % 通道 31 (过阻尼): 保持原样
    Weights_31.Q = 0.7;
    Weights_31.Ki = 2.4;
    Weights_31.R = 0.1;
    
    % 通道 32 (欠阻尼): R 值将在后续代码中根据误差动态重写
    Weights_32.Q = 1.8;   
    Weights_32.Ki = 6.3;
    Weights_32.R = 0.0; % 初始值，会被覆盖

    % 稳态死区
    Err_Band_31 = 0.2; 
    Err_Band_32 = 0.2;

    % ==========================================================
    %       通道 31 (Channel 31)
    % ==========================================================
    [A31, B31] = GetStateSpace(X31_num, X31_den, K31, Ratio, Tp31, dt);
    
    [model_31, Y_fast_31] = UpdateFastModel_StateSpace(model_31, u_prev_31, A31, B31);
    [delay_buffer_31, head_31, Y_delayed_31] = UpdateDelayBuffer(delay_buffer_31, head_31, Y_fast_31, Tau31, dt, MAX_BUF);
    
    pred_error_31 = Q31Real - Y_delayed_31;
    Target_31 = Q31Ref - pred_error_31;
    
    err_fast_31 = Target_31 - Y_fast_31;
    
    if u_prev_31 > 0 && u_prev_31 < 100
        x_int_31 = x_int_31 + err_fast_31 * dt;
    else
        if (u_prev_31 >= 100 && err_fast_31 < 0) || (u_prev_31 <= 0 && err_fast_31 > 0)
             x_int_31 = x_int_31 + err_fast_31 * dt;
        end
    end

    x0_aug_31 = [model_31; x_int_31];
    real_err_31 = Q31Ref - Q31Real;
    
    if abs(real_err_31) < Err_Band_31
        u_raw_31 = u_prev_31;
    else
        [u_raw_31, u_opt_guess_31] = Run_iLQR_Augmented(x0_aug_31, Target_31, u_prev_31, ...
                                                        A31, B31, Weights_31, u_opt_guess_31, HORIZON, dt);
    end

    Gap_31 = 1.4; 
    V31 = InverseDeadzoneComp_Soft(u_raw_31, u_prev_31, Gap_31, real_err_31, 1.5);
    u_prev_31 = V31;

    % ==========================================================
    %       通道 32 (Channel 32)
    % ==========================================================
    [A32, B32] = GetStateSpace(X32_num, X32_den, K32, Ratio, Tp32, dt);
    
    [model_32, Y_fast_32] = UpdateFastModel_StateSpace(model_32, u_prev_32, A32, B32);
    [delay_buffer_32, head_32, Y_delayed_32] = UpdateDelayBuffer(delay_buffer_32, head_32, Y_fast_32, Tau32, dt, MAX_BUF);
    
    pred_error_32 = Q32Real - Y_delayed_32;
    Target_32 = Q32Ref - pred_error_32;

    err_fast_32 = Target_32 - Y_fast_32;
    
    if u_prev_32 > 0 && u_prev_32 < 100
        x_int_32 = x_int_32 + err_fast_32 * dt;
    else
         if (u_prev_32 >= 100 && err_fast_32 < 0) || (u_prev_32 <= 0 && err_fast_32 > 0)
             x_int_32 = x_int_32 + err_fast_32 * dt;
         end
    end

    x0_aug_32 = [model_32; x_int_32];
    real_err_32 = Q32Ref - Q32Real;

    % === [新增逻辑] 32路 自适应 R 权重调整 ===
    % 策略：大误差 -> 松刹车 (R小)；小误差 -> 踩死刹车 (R大)
    Adaptive_Threshold_32 = 20; % 误差分界线 (可根据实际情况微调)
    
    if abs(real_err_32) > Adaptive_Threshold_32
        % 误差大：关闭阻尼，全速响应
        Weights_32.R = 0.00; 
    else
        % 误差小：开启强阻尼，抑制震荡
        % R = 20.0 是一个非常强的值，能有效按住阀门
        Weights_32.R = 0.035; 
    end

    % 运行优化器
    if abs(real_err_32) < Err_Band_32
        u_raw_32 = u_prev_32;
    else
        [u_raw_32, u_opt_guess_32] = Run_iLQR_Augmented(x0_aug_32, Target_32, u_prev_32, ...
                                                        A32, B32, Weights_32, u_opt_guess_32, HORIZON, dt);
    end

    Gap_32 = 0.6;
    V32 = InverseDeadzoneComp_Soft(u_raw_32, u_prev_32, Gap_32, real_err_32, 0.5);
    u_prev_32 = V32;
end

%% === 核心模块: 增广 iLQR 优化器 ===
function [u_optimal, u_guess_next] = Run_iLQR_Augmented(x0_aug, Ref, u_last, A_phys, B_phys, W, u_guess, N, dt)
    C_phys = [0, 0, 1]; 
    Aa = [A_phys, zeros(3,1); -C_phys*dt, 1];
    Ba = [B_phys; 0];

    Q_cost = W.Q;
    R_cost = W.R;
    Ki_cost = W.Ki; 
    
    alpha = 0.15; 
    max_iter = 5; 

    U = [u_guess(2:end); u_guess(end)]; 
    
    for iter = 1:max_iter
        X_traj = zeros(4, N+1); 
        X_traj(:, 1) = x0_aug;
        for k = 1:N
            x_next = Aa * X_traj(:, k) + Ba * U(k);
            x_next(4) = x_next(4) + Ref * dt;
            X_traj(:, k+1) = x_next;
        end
        
        delta_J_U = zeros(N, 1);
        lambda = zeros(4, 1); 
        u_prev_step = u_last;
        
        for k = N:-1:1
            x_curr = X_traj(:, k+1);
            y_curr = C_phys * x_curr(1:3); 
            int_curr = x_curr(4);          
            
            if k > 1, u_act = U(k); u_prev_act = U(k-1);
            else, u_act = U(k); u_prev_act = u_prev_step; end
            
            grad_x_phys = 2 * Q_cost * C_phys' * (y_curr - Ref);
            grad_x_int = 2 * Ki_cost * int_curr;
            grad_x_aug = [grad_x_phys; grad_x_int];
            
            lambda = Aa' * lambda + grad_x_aug;
            
            grad_u_smooth = 2 * R_cost * (u_act - u_prev_act);
            delta_J_U(k) = Ba' * lambda + grad_u_smooth;
        end
        
        U = U - alpha * delta_J_U;
        U = max(0, min(100, U));
    end
    u_optimal = U(1);       
    u_guess_next = U;       
end

%% === 辅助模块 ===
function [A, B] = GetStateSpace(num, den, K, Ratio, Tp, Ts)
    wn2 = den(3); zw = den(2); K_valve = num; K_total = K * Ratio;
    A = [1, Ts, 0; -wn2*Ts, 1 - zw*Ts, 0; K_total*Ts/max(Tp,0.1), 0, 1 - Ts/max(Tp,0.1)];
    B = [0; K_valve * Ts; 0];
end

function [state_new, y_out] = UpdateFastModel_StateSpace(state, u, A, B)
    state_new = A * state + B * u;
    y_out = state_new(3); 
end

function [buffer, head_idx, y_delayed] = UpdateDelayBuffer(buffer, head, y_in, Tau, Ts, MAX_BUF)
    delay_steps = round(Tau / Ts);
    delay_steps = max(1, min(delay_steps, MAX_BUF - 1));
    buffer(head) = y_in;
    read_idx = head - delay_steps;
    if read_idx < 1, read_idx = read_idx + MAX_BUF; end
    y_delayed = buffer(read_idx);
    head_idx = head + 1;
    if head_idx > MAX_BUF, head_idx = 1; end
end

function Ratio = CalculateFlowRatio(P30, T30, P_ref, T_ref, R_gas, Patm)
    Tk_dyn = T30 + 273.15; delta_P_dyn = P30 - Patm;
    if delta_P_dyn < 0, delta_P_dyn = 0; end
    Term_Dyn = sqrt((P30 * 1000 * delta_P_dyn * 1000) / (R_gas * Tk_dyn));
    Tk_ref = T_ref + 273.15; delta_P_ref = P_ref - Patm;
    if delta_P_ref < 0, delta_P_ref = 0; end
    Term_Ref = sqrt((P_ref * 1000 * delta_P_ref * 1000) / (R_gas * Tk_ref));
    if Term_Ref < 1e-6, Ratio = 1; else, Ratio = max(Term_Dyn / Term_Ref, 0.05); end
end

function u_final = InverseDeadzoneComp_Soft(u_cmd, u_last, gap, error, err_threshold)
    delta = u_cmd - u_last;
    alpha = min(abs(error) / err_threshold, 1.0);
    real_gap = gap * alpha;
    Noise_Threshold = 0.02; 
    if abs(delta) > Noise_Threshold 
        if delta > 0, u_final = u_cmd + real_gap; else, u_final = u_cmd - real_gap; end
    else, u_final = u_last; end
    u_final = max(0, min(100, u_final));
end
